simulink model "Panneau_PV_avec_charge"  (R2017b)
settings: Solver=VariableStepAuto  StartTime=0.0  StopTime=3600*24  RelTol=1e-3
libraries: fl_lib x9, nesl_utility x8, elec_lib x6, Library_SII x2
settings Model: Creator=Cedrick  LastModifiedBy=Cedrick

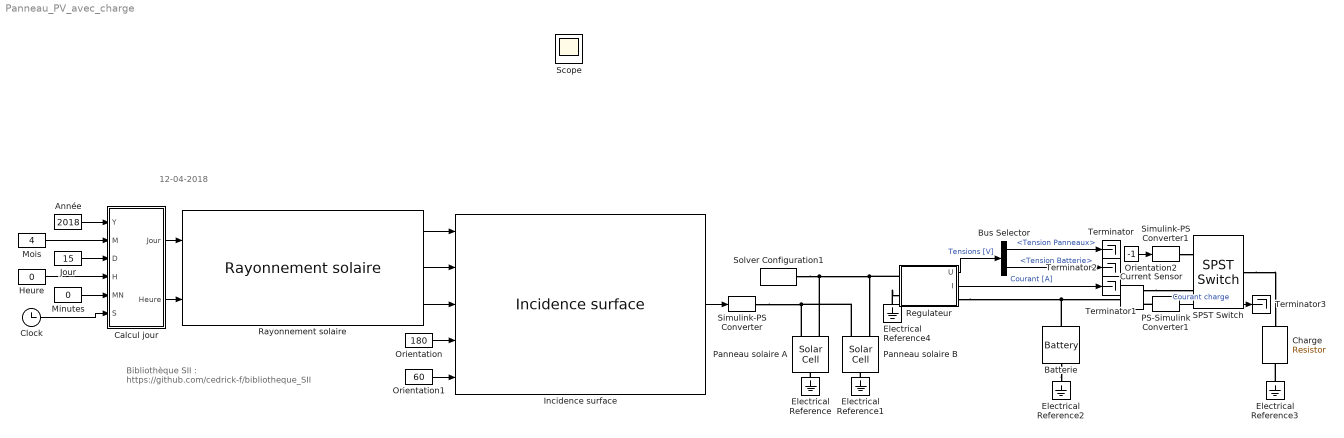
== system Panneau_PV_avec_charge ==
  note: 12-04-2018
  note: Bibliothèque SII :
      | https://github.com/cedrick-f/bibliotheque_SII
  Année : Constant  Value=2018
  Batterie : elec_lib/Sources/Battery  Vnom=12 V  R1=2 Ohm  prm_AH=2  AH=12 hr*A  V1=11.5 V  AH1=6 hr*A  prm_R2=2  R2=2000 Ohm  prm_fade=1  N_fade=100  AH_fade=45 hr*A  R1_fade=2.02 Ohm  V1_fade=10.35 V  i_specify=off  i_priority=None  i=0 A  i_nominal_specify=off  i_nominal_unit=A  i_nominal_value=1  v_specify=on  v_priority=None  v=12 V  v_nominal_specify=off  v_nominal_unit=V  v_nominal_value=1  charge_specify=on  charge_priority=High  charge=12 hr*A  charge_nominal_specify=off  charge_nominal_unit=hr*A  charge_nominal_value=1  num_cycles_specify=off  num_cycles_priority=High  num_cycles=0  num_cycles_nominal_specify=off  num_cycles_nominal_unit=1  num_cycles_nominal_value=1  thermal_mass=30000 J/K  Tmeas=298.15 K  Vnom_T2=12 V  R1_T2=2.2 Ohm  V1_T2=11.4 V  R2_T2=2200 Ohm  Tmeas2=273.15 K  temperature_specify=off  temperature_priority=High  temperature=298.15 K  temperature_nominal_specify=off  temperature_nominal_unit=K  temperature_nominal_value=1
      settings: SourceProductName=Simscape Electronics  SourceProductBaseCode=SN
      settings: AttributesFormatString=|
      | %<Vnom> V
      | %<AH> Ah
  Bus Selector : BusSelector  OutputSignals=Tension Panneaux,Tension Batterie
  Calcul jour : MATLAB Function  TreatAsAtomicUnit=on
  Charge : elec_lib/Passive Devices/Resistor  R=3 Ohm  R_tol=5  enable_R_tol=0  tol_distribution=1  nSigma=4  enable_operating_limits=0  operating_limit_action=2  max_working_voltage=100 V  power_rating=1 W  enable_faults=0  fault_action=1  R_faulted=inf Ohm  enable_temporal_fault=0  t_fault=1 s  enable_behavioral_fault=0  max_permissible_current=1 A  t_fail_on_current=1 s  noise_mode=0  sample_time=1e-3 s  repeatability=1  auto_seed=585372041  user_seed=0  Tdevice=25 degC  alpha=3.93e-3 1/K  Tmeas=25 degC  thermal_mass=100 J/K  power_derating_T1=70 degC  power_derating_T2=155 degC  operating_temperature_range_vec=[-50, 150] degC  temperature_specify=off  temperature_priority=High  temperature=298.15 K  temperature_nominal_specify=off  temperature_nominal_unit=K  temperature_nominal_value=1
      settings: AttributesFormatString=%<R> Ohm
  Clock : Clock
  Current Sensor : fl_lib/Electrical/Electrical Sensors/Current Sensor
  Electrical Reference{,1..4} (5 alike) : fl_lib/Electrical/Electrical Elements/Electrical Reference
  Heure : Constant  Value=0
  Incidence surface : Library_SII/Thermique/Incidence surface  lat=[45 46 46]  lon=[-3 05 10]  T_air=20  Hr=0.5  P_Atm=98232  B=0.1
      settings: SourceProductName=SII
  Jour : Constant  Value=15
  Minutes : Constant  Value=0
  Mois : Constant  Value=4
  Orientation : Constant  Value=180
  Orientation1 : Constant  Value=60
  Orientation2 : Constant  Value=-1
  PS-Simulink Converter1 : nesl_utility/PS-Simulink Converter  PhysicalDomain=network_engine_domain  SubClassName=ps_output  LeftPortType=input  RightPortType=output  PseudoPeriodic=off  Frequencies=[]  Unit=1  AffineConversion=off
  Panneau solaire A : elec_lib/Sources/Solar Cell  prm=1  Isc=7.34 A  Voc=0.6 V  Is=1e-6 A  Is2=0 A  Iph=7.34 A  Ir0=1000 W/m^2  ec=1.5  N2=2  Rs=0 Ohm  Rp=inf Ohm  N_series=36  TIPH1=0 1/K  EG=1.11 eV  TXIS1=3  TXIS2=3  TRS1=0  TRP1=0  Tmeas=25 degC  TFIXED=25 degC  thermal_mass=100 J/K  initial_temperature=25 degC
      settings: AttributesFormatString=%<N_series> cellules  SourceProductName=Simscape Electronics  SourceProductBaseCode=SN
  Panneau solaire B : elec_lib/Sources/Solar Cell  prm=1  Isc=7.34 A  Voc=0.6 V  Is=1e-6 A  Is2=0 A  Iph=7.34 A  Ir0=1000 W/m^2  ec=1.5  N2=2  Rs=0 Ohm  Rp=inf Ohm  N_series=36  TIPH1=0 1/K  EG=1.11 eV  TXIS1=3  TXIS2=3  TRS1=0  TRP1=0  Tmeas=25 degC  TFIXED=25 degC  thermal_mass=100 J/K  initial_temperature=25 degC
      settings: AttributesFormatString=%<N_series> cellules  SourceProductName=Simscape Electronics  SourceProductBaseCode=SN
  Rayonnement solaire : Library_SII/Thermique/Rayonnement solaire  lat=[45 46 46]  lon=[-3 05 10]  T_air=20  Hr=0.5  P_Atm=98232  B=0.1
      settings: SourceProductName=SII
  Regulateur : Subsystem
  SPST Switch : elec_lib/Passive Devices/Switches/SPST Switch  R_closed=0.01 Ohm  G_open=1e-6 S  Threshold=0 V  Width=0 V  model_dynamics=0  t_on=1e-3 s  t_off=1e-3 s  initial_vT=0 V
      settings: SourceProductName=Simscape Electronics  SourceProductBaseCode=SN
  Simulink-PS Converter : nesl_utility/Simulink-PS Converter  PhysicalDomain=network_engine_domain  SubClassName=ps_input  LeftPortType=input  RightPortType=output  PseudoPeriodic=off  Frequencies=[]  NoiseDistribution=none  NoiseParameters=[]  Unit=1  AffineConversion=off  FilteringAndDerivatives=provide  SimscapeFilterOrder=1  InputFilterTimeConstant=0.001  UdotUserProvided=0
  Simulink-PS Converter1 : nesl_utility/Simulink-PS Converter  PhysicalDomain=network_engine_domain  SubClassName=ps_input  LeftPortType=input  RightPortType=output  PseudoPeriodic=off  Frequencies=[]  NoiseDistribution=none  NoiseParameters=[]  Unit=1  AffineConversion=off  FilteringAndDerivatives=provide  SimscapeFilterOrder=1  InputFilterTimeConstant=0.001  UdotUserProvided=0
  Solver Configuration1 : nesl_utility/Solver Configuration  PhysicalDomain=network_engine_domain  SubClassName=solver  LeftPortType=input  RightPortType=generic  Accelerate=off  Tones=[]  Harmonics=[]  SimulateNoise=off  Profile=off  UseLocalSampling=off  EnableSwitchedLinearOptims=on  FrequencyDomain=off  UseCCode=off  RelTol=0.001  AbsTol=1e-06  MinStep=1e-09  ToWorkspace=off  RevertToSquareIcSolve=off  NumHomotopyIterations=100  PhasorMode=off  PhasorModeNumHarmonics=1  DoDC=off  ResidualTolerance=1e-09  UseLocalSolver=off  LocalSolverChoice=NE_BACKWARD_EULER_ADVANCER  LocalSolverSampleTime=0.001  DoFixedCost=off  MaxNonlinIter=3  MaxModeIter=2  LinearAlgebra=Sparse  DelaysMemoryBudget=1024  AutomaticFiltering=on  FilteringTimeConstant=0.001
  Terminator{,1..3} (4 alike) : Terminator
  Scope : Scope
  wires:
  Rayonnement solaire/2 -> Incidence surface/2
  Rayonnement solaire/3 -> Incidence surface/3
  Rayonnement solaire/1 -> Incidence surface/1
  Incidence surface/1 -> Simulink-PS Converter/1
  Année/1 -> Calcul jour/1(Y)
  Clock/1 -> Calcul jour/6(S)
  Mois/1 -> Calcul jour/2(M)
  Jour/1 -> Calcul jour/3(D)
  Calcul jour/1(Jour) -> Rayonnement solaire/1
  Calcul jour/2(Heure) -> Rayonnement solaire/2
  Heure/1 -> Calcul jour/4(H)
  Minutes/1 -> Calcul jour/5(MN)
  Orientation/1 -> Incidence surface/4
  Orientation1/1 -> Incidence surface/5
  Orientation2/1 -> Simulink-PS Converter1/1
  Regulateur/1(U) -> Bus Selector/1  "Tensions [V]"
  Regulateur/2(I) -> Terminator1/1  "Courant [A]"
  Bus Selector/2 -> Terminator2/1  "<Tension Batterie>"
  Bus Selector/1 -> Terminator/1  "<Tension Panneaux>"
  PS-Simulink Converter1/1 -> Terminator3/1  "Courant charge"
  connections:
  Simulink-PS Converter/RConn1 -- Panneau solaire A/LConn1 -- Panneau solaire B/LConn1
  Solver Configuration1/RConn1 -- Regulateur/LConn1 -- Panneau solaire B/LConn2 -- Panneau solaire A/LConn2
  Electrical Reference/LConn1 -- Panneau solaire A/RConn1
  Electrical Reference1/LConn1 -- Panneau solaire B/RConn1
  Batterie/RConn1 -- Electrical Reference2/LConn1
  Electrical Reference3/LConn1 -- Charge/RConn1
  Simulink-PS Converter1/RConn1 -- SPST Switch/LConn1
  SPST Switch/RConn1 -- Charge/LConn1
  Batterie/LConn1 -- Regulateur/RConn1 -- Current Sensor/LConn1
  Electrical Reference4/LConn1 -- Regulateur/LConn2
  PS-Simulink Converter1/LConn1 -- Current Sensor/RConn1
  Current Sensor/RConn2 -- SPST Switch/LConn2

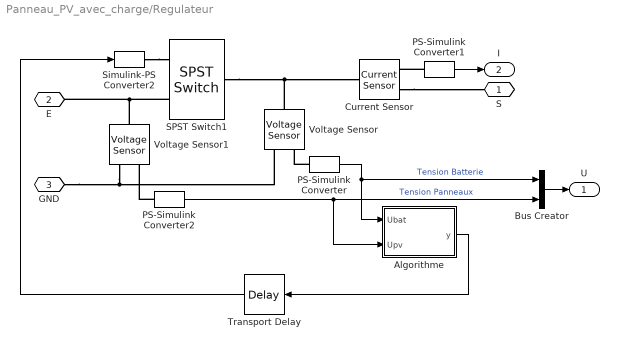
== system Panneau_PV_avec_charge/Regulateur ==
  Algorithme : MATLAB Function  TreatAsAtomicUnit=on
      settings: MinAlgLoopOccurrences=on
  Bus Creator : BusCreator  Inputs=2
  Current Sensor : fl_lib/Electrical/Electrical Sensors/Current Sensor
  PS-Simulink Converter : nesl_utility/PS-Simulink Converter  PhysicalDomain=network_engine_domain  SubClassName=ps_output  LeftPortType=input  RightPortType=output  PseudoPeriodic=off  Frequencies=[]  Unit=1  AffineConversion=off
  PS-Simulink Converter1 : nesl_utility/PS-Simulink Converter  PhysicalDomain=network_engine_domain  SubClassName=ps_output  LeftPortType=input  RightPortType=output  PseudoPeriodic=off  Frequencies=[]  Unit=1  AffineConversion=off
  PS-Simulink Converter2 : nesl_utility/PS-Simulink Converter  PhysicalDomain=network_engine_domain  SubClassName=ps_output  LeftPortType=input  RightPortType=output  PseudoPeriodic=off  Frequencies=[]  Unit=1  AffineConversion=off
  SPST Switch1 : elec_lib/Passive Devices/Switches/SPST Switch  R_closed=0.01 Ohm  G_open=1e-6 S  Threshold=0 V  Width=0 V  model_dynamics=0  t_on=1e-3 s  t_off=1e-3 s  initial_vT=0 V
      settings: SourceProductName=Simscape Electronics  SourceProductBaseCode=SN
  Simulink-PS Converter2 : nesl_utility/Simulink-PS Converter  PhysicalDomain=network_engine_domain  SubClassName=ps_input  LeftPortType=input  RightPortType=output  PseudoPeriodic=off  Frequencies=[]  NoiseDistribution=none  NoiseParameters=[]  Unit=1  AffineConversion=off  FilteringAndDerivatives=provide  SimscapeFilterOrder=1  InputFilterTimeConstant=0.001  UdotUserProvided=0
  Transport Delay : TransportDelay
  Voltage Sensor : fl_lib/Electrical/Electrical Sensors/Voltage Sensor
  Voltage Sensor1 : fl_lib/Electrical/Electrical Sensors/Voltage Sensor
  S : PMIOPort  Port=1  Side=Right
  E : PMIOPort  Port=2  Side=Left
  GND : PMIOPort  Port=3  Side=Left
  U : Outport
  I : Outport  Port=2
  wires:
  PS-Simulink Converter1/1 -> I/1
  PS-Simulink Converter/1 -> Algorithme/1(Ubat), Bus Creator/1  "Tension Batterie"
  Algorithme/1(y) -> Transport Delay/1
  PS-Simulink Converter2/1 -> Algorithme/2(Upv), Bus Creator/2  "Tension Panneaux"
  Bus Creator/1 -> U/1
  Transport Delay/1 -> Simulink-PS Converter2/1
  connections:
  Simulink-PS Converter2/RConn1 -- SPST Switch1/LConn1
  SPST Switch1/RConn1 -- Voltage Sensor/LConn1 -- Current Sensor/LConn1
  SPST Switch1/LConn2 -- Voltage Sensor1/LConn1 -- E/RConn1
  GND/RConn1 -- Voltage Sensor/RConn2 -- Voltage Sensor1/RConn2
  PS-Simulink Converter/LConn1 -- Voltage Sensor/RConn1
  Current Sensor/RConn2 -- S/RConn1
  PS-Simulink Converter1/LConn1 -- Current Sensor/RConn1
  PS-Simulink Converter2/LConn1 -- Voltage Sensor1/RConn1

== matlab function Panneau_PV_avec_charge/Regulateur/Algorithme ==
  data: Ubat input; y output; Upv input
function y = fcn(Ubat,Upv)

Uref = 13.6; %V
DeltaU = 0.4; %V

if Ubat > Uref
    y = -1; % Circuit ouvert
else
    if Upv-Ubat > DeltaU
        y = 1;  % Circuit fermé
    else
        y = -1; % Circuit ouvert
    end
end

== matlab function Panneau_PV_avec_charge/Calcul jour ==
  data: Y input; Jour output; M input; D input; H input; MN input; S input; Heure output
function [Jour, Heure]= fcn(Y,M,D,H,MN,S)

coder.extrinsic('datenum'); 
j1 = 1;
j2 = 1;
[j1] = datenum(Y,M,D);
[j2] = datenum(Y,1,1);
Jour = j1 - j2 + 1;

Heure = H*3600+MN*60+S;
